simulink model "RCK_Model"  (R2016b)
settings: Solver=VariableStepAuto  StartTime=0.0  StopTime=500  RelTol=1e-3  EnableMultiTasking=on
PreLoadFcn:
  | defineRCKParams
undefined symbols (not defined in the file): params
settings Model: Creator=kdeeley  LastModifiedBy=kdeeley
settings DataIOCC: LimitDataPoints=on  SaveFormat=Array
settings OptimizationCC: LifeSpan=inf
settings DebuggingCC: AllowSymbolicDim=off  SFUnexpectedBacktrackingDiag=warning  SFNoUnconditionalDefaultTransitionDiag=warning  SFUnconditionalPathOutOfParentDiag=warning  SFExecutionAtInitializationDiag=none  SFUnreachableStateOrJunctionDiag=warning  SFDanglingTransitionDiag=warning
settings ModelReferenceCC: PropagateSignalLabelsOutOfModel=off
settings CodeAppCC: CustomSymbolStrSimulinkFcn=$N
settings GRTTargetCC: TargetLangStandard=C89/C90 (ANSI)
settings ConfigComp: CovMetricSettings=dw  CovHtmlReporting=on  CovSaveCumulativeToWorkspaceVar=on  CovSaveSingleToWorkspaceVar=on  CovExternalEMLEnable=off

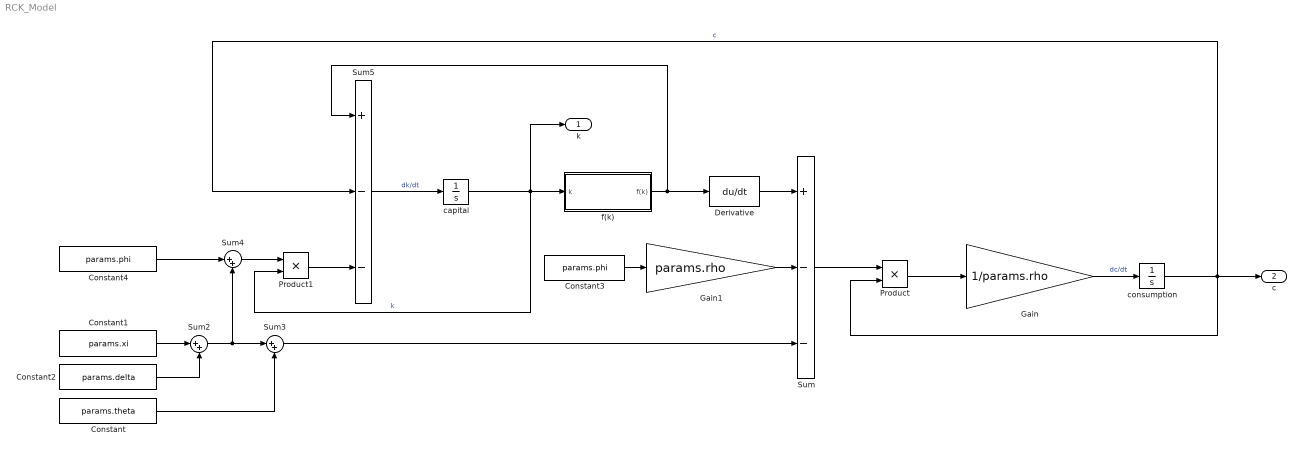
== system RCK_Model ==
  Constant : Constant  Value=params.theta
  Constant1 : Constant  Value=params.xi
  Constant2 : Constant  Value=params.delta
  Constant3 : Constant  Value=params.phi
  Constant4 : Constant  Value=params.phi
  Derivative : Derivative
  Gain : Gain  Gain=1/params.rho
  Gain1 : Gain  Gain=params.rho
  Product : Product
  Product1 : Product
  Sum : Sum  Inputs=+--
  Sum2 : Sum  Inputs=|++
  Sum3 : Sum  Inputs=|++
  Sum4 : Sum  Inputs=|++
  Sum5 : Sum  Inputs=+--
  capital : Integrator  InitialCondition=params.k0
  consumption : Integrator  InitialCondition=params.c0
  f(k) : Subsystem
  k : Outport
  c : Outport  Port=2
  wires:
  Gain/1 -> consumption/1  "dc/dt"
  consumption/1 -> Product/2, c/1, Sum5/2  "c"
  Sum/1 -> Product/1
  Product/1 -> Gain/1
  Sum5/1 -> capital/1  "dk/dt"
  f(k)/1(f(k)) -> Sum5/1, Derivative/1
  Constant3/1 -> Gain1/1
  Constant2/1 -> Sum2/2
  Sum2/1 -> Sum3/1, Sum4/2
  Constant/1 -> Sum3/2
  Sum3/1 -> Sum/3
  Gain1/1 -> Sum/2
  Product1/1 -> Sum5/3
  capital/1 -> Product1/2, k/1, f(k)/1(k)  "k"
  Sum4/1 -> Product1/1
  Constant4/1 -> Sum4/1
  Constant1/1 -> Sum2/1
  Derivative/1 -> Sum/1

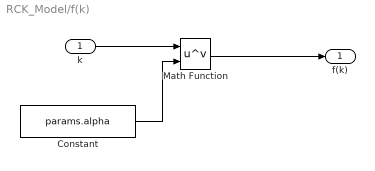
== system RCK_Model/f(k) ==
  k : Inport
  Constant : Constant  Value=params.alpha
  Math Function : Math  Operator=pow  SaturateOnIntegerOverflow=on
  f(k) : Outport
  wires:
  k/1 -> Math Function/1
  Constant/1 -> Math Function/2
  Math Function/1 -> f(k)/1
